simulink library "M160_control_lib"  (Simulink 7.8)
settings: Solver=FixedStepDiscrete  StartTime=0.0  StopTime=10.0  RelTol=1e-3
PreLoadFcn:
  | update_path
undefined symbols (not defined in the file): Egc_tiTEgasFilt, ehooks_medc17flex_devlib_io_block, Fmc_facKFuelMassCorr, Fmc_tiTFuelMassCorr, Itc_rpmEngSpdHyst, Itc_rpmEngSpdMax, Tvc_facDutycyclePIDLimitMax, Tvc_facDutycyclePIDLimitMin, Tvc_facKDutycycle, Tvc_tiTnDutycycle, Tvc_tiTvDutycycle
libraries: simulink x6
(part 2 of 2)

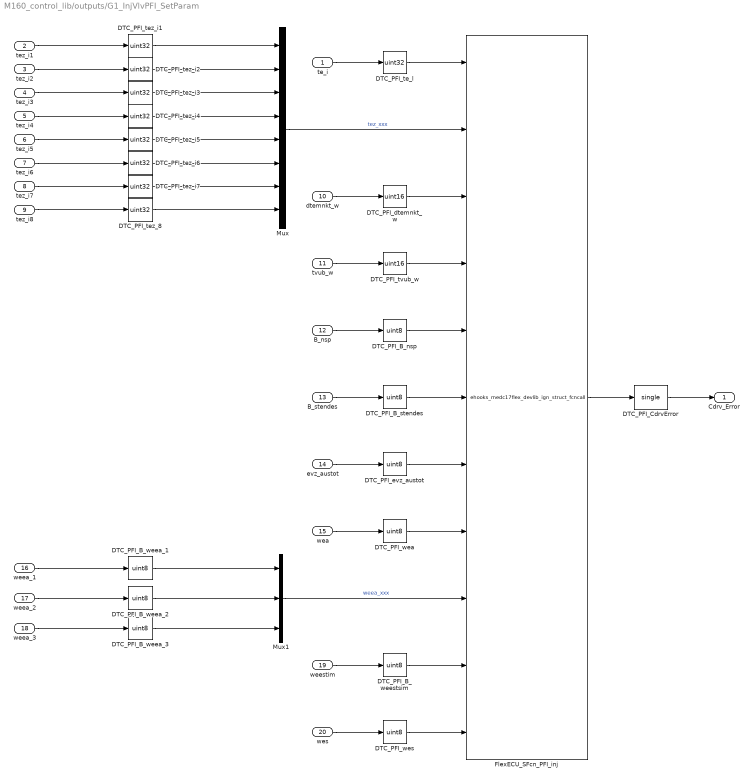
== system M160_control_lib/outputs/G1_InjVlvPFI_SetParam ==
  te_i : Inport
  tez_i1 : Inport  Port=2
  tez_i2 : Inport  Port=3
  tez_i3 : Inport  Port=4
  tez_i4 : Inport  Port=5
  tez_i5 : Inport  Port=6
  tez_i6 : Inport  Port=7
  tez_i7 : Inport  Port=8
  tez_i8 : Inport  Port=9
  dtemnkt_w : Inport  Port=10
  tvub_w : Inport  Port=11
  B_nsp : Inport  Port=12
  B_stendes : Inport  Port=13
  evz_austot : Inport  Port=14
  wea : Inport  Port=15
  weea_1 : Inport  Port=16
  weea_2 : Inport  Port=17
  weea_3 : Inport  Port=18
  weestim : Inport  Port=19
  wes : Inport  Port=20
  DTC_PFI_B_nsp : DataTypeConversion  OutDataTypeStr=uint8  RndMeth=Nearest
  DTC_PFI_B_stendes : DataTypeConversion  OutDataTypeStr=uint8  RndMeth=Nearest
  DTC_PFI_B_weea_1 : DataTypeConversion  OutDataTypeStr=uint8  RndMeth=Nearest
  DTC_PFI_B_weea_2 : DataTypeConversion  OutDataTypeStr=uint8
  DTC_PFI_B_weea_3 : DataTypeConversion  OutDataTypeStr=uint8  RndMeth=Nearest
  DTC_PFI_B_weestsim : DataTypeConversion  OutDataTypeStr=uint8  RndMeth=Nearest
  DTC_PFI_CdrvError : DataTypeConversion  OutDataTypeStr=single
  DTC_PFI_dtemnkt_w : DataTypeConversion  OutDataTypeStr=uint16  RndMeth=Nearest
  DTC_PFI_evz_austot : DataTypeConversion  OutDataTypeStr=uint8  RndMeth=Nearest
  DTC_PFI_te_l : DataTypeConversion  OutDataTypeStr=uint32  RndMeth=Nearest
  DTC_PFI_tez_8 : DataTypeConversion  OutDataTypeStr=uint32  RndMeth=Nearest
  DTC_PFI_tez_i{1..7} (7 alike) : DataTypeConversion  OutDataTypeStr=uint32  RndMeth=Nearest
  DTC_PFI_tvub_w : DataTypeConversion  OutDataTypeStr=uint16  RndMeth=Nearest
  DTC_PFI_wea : DataTypeConversion  OutDataTypeStr=uint8  RndMeth=Nearest
  DTC_PFI_wes : DataTypeConversion  OutDataTypeStr=uint8  RndMeth=Nearest
  FlexECU_SFcn_PFI_inj : S-Function  FunctionName=ehooks_medc17flex_devlib_ign_struct_fcncall  Parameters=NoInputPorts, NoOutputPorts, InputPortDataTypes, OutputPortDataTypes, CFunctionArgTypes, CFunctionName, StructMemberNames, StructTypeName, InputPortDataWidths, OutputPortDataWidths  EnableBusSupport=off  mask{NoInputPorts=11, NoOutputPorts=1, InputPortDataTypes=uint32, uint32, uint16, uint16,uint8,uint8,uint8,uint8,uint8,uint8,uint8, OutputPortDataTypes=uint8, CFunctionArgTypes=ret,val, refin, val,val,val,val,val, val, refin, val, val, CFunctionName=InjVlvPfi_SetParam, StructMemberNames=te_l,  tez_l, dtemnkt_w, tvub_w, B_nsp, B_stendes, evz_austot, wea, weea, weestsim, wes, StructTypeName=InjVlvPfiInterface_type, InputPortDataWidths=1,8,1,1,1,1,1,1,3,1,1, OutputPortDataWidths=1}
      mask prompts: NoInputPorts "Number of input ports"; NoOutputPorts "Number of output ports"; InputPortDataTypes "Input port data types"; OutputPortDataTypes "Output port data types"; CFunctionArgTypes "C function argument types"; CFunctionName "C function name"; StructMemberNames "Structure member names"; StructTypeName "Structure type name"; InputPortDataWidths "Input port widths"; OutputPortDataWidths "Output port widths"
      mask Display: disp('EHOOKS FlexECU\nDevLib Wrapper\nS-Function')
  Mux : Mux  Inputs=8
  Mux1 : Mux  Inputs=3
  Cdrv_Error : Outport
  wires:
  DTC_PFI_CdrvError/1 -> Cdrv_Error/1
  FlexECU_SFcn_PFI_inj/1 -> DTC_PFI_CdrvError/1
  DTC_PFI_B_stendes/1 -> FlexECU_SFcn_PFI_inj/6
  B_stendes/1 -> DTC_PFI_B_stendes/1
  DTC_PFI_B_nsp/1 -> FlexECU_SFcn_PFI_inj/5
  B_nsp/1 -> DTC_PFI_B_nsp/1
  DTC_PFI_tvub_w/1 -> FlexECU_SFcn_PFI_inj/4
  tvub_w/1 -> DTC_PFI_tvub_w/1
  DTC_PFI_dtemnkt_w/1 -> FlexECU_SFcn_PFI_inj/3
  dtemnkt_w/1 -> DTC_PFI_dtemnkt_w/1
  te_i/1 -> DTC_PFI_te_l/1
  DTC_PFI_evz_austot/1 -> FlexECU_SFcn_PFI_inj/7
  DTC_PFI_wea/1 -> FlexECU_SFcn_PFI_inj/8
  DTC_PFI_B_weestsim/1 -> FlexECU_SFcn_PFI_inj/10
  DTC_PFI_wes/1 -> FlexECU_SFcn_PFI_inj/11
  evz_austot/1 -> DTC_PFI_evz_austot/1
  wea/1 -> DTC_PFI_wea/1
  weea_1/1 -> DTC_PFI_B_weea_1/1
  weestim/1 -> DTC_PFI_B_weestsim/1
  wes/1 -> DTC_PFI_wes/1
  DTC_PFI_te_l/1 -> FlexECU_SFcn_PFI_inj/1
  tez_i1/1 -> DTC_PFI_tez_i1/1
  tez_i2/1 -> DTC_PFI_tez_i2/1
  tez_i3/1 -> DTC_PFI_tez_i3/1
  tez_i4/1 -> DTC_PFI_tez_i4/1
  tez_i5/1 -> DTC_PFI_tez_i5/1
  tez_i6/1 -> DTC_PFI_tez_i6/1
  tez_i7/1 -> DTC_PFI_tez_i7/1
  tez_i8/1 -> DTC_PFI_tez_8/1
  DTC_PFI_tez_i1/1 -> Mux/1
  DTC_PFI_tez_i2/1 -> Mux/2
  DTC_PFI_tez_i3/1 -> Mux/3
  DTC_PFI_tez_i4/1 -> Mux/4
  DTC_PFI_tez_i5/1 -> Mux/5
  DTC_PFI_tez_i6/1 -> Mux/6
  DTC_PFI_tez_i7/1 -> Mux/7
  DTC_PFI_tez_8/1 -> Mux/8
  Mux/1 -> FlexECU_SFcn_PFI_inj/2  "tez_xxx"
  weea_2/1 -> DTC_PFI_B_weea_2/1
  weea_3/1 -> DTC_PFI_B_weea_3/1
  DTC_PFI_B_weea_1/1 -> Mux1/1
  DTC_PFI_B_weea_2/1 -> Mux1/2
  DTC_PFI_B_weea_3/1 -> Mux1/3
  Mux1/1 -> FlexECU_SFcn_PFI_inj/9  "weea_xxx"

== system M160_control_lib/outputs/G1_Inj_Set_DEVE_forPFI ==
  B_desee : Inport
  B_sa : Inport  Port=2
  DTC_PFI_DEVE_Bdesee : DataTypeConversion  OutDataTypeStr=uint8  RndMeth=Nearest
  DTC_PFI_DEVE_Bsa : DataTypeConversion  OutDataTypeStr=uint8  RndMeth=Nearest
  DTC_PFI_DEVE_Bsa1 : DataTypeConversion  OutDataTypeStr=single
  FlexECU_SFcn_PFI_inj : S-Function  FunctionName=ehooks_medc17flex_devlib_ign_struct_fcncall  Parameters=NoInputPorts, NoOutputPorts, InputPortDataTypes, OutputPortDataTypes, CFunctionArgTypes, CFunctionName, StructMemberNames, StructTypeName, InputPortDataWidths, OutputPortDataWidths  EnableBusSupport=off  mask{NoInputPorts=2, NoOutputPorts=1, InputPortDataTypes=uint8,uint8, OutputPortDataTypes=uint8, CFunctionArgTypes=ret, val, val, CFunctionName=InjVlvDeve_SetParam, StructMemberNames=B_desee, B_sa, StructTypeName=InjVlvDeveInterface_type, InputPortDataWidths=1,1, OutputPortDataWidths=1}
      mask prompts: NoInputPorts "Number of input ports"; NoOutputPorts "Number of output ports"; InputPortDataTypes "Input port data types"; OutputPortDataTypes "Output port data types"; CFunctionArgTypes "C function argument types"; CFunctionName "C function name"; StructMemberNames "Structure member names"; StructTypeName "Structure type name"; InputPortDataWidths "Input port widths"; OutputPortDataWidths "Output port widths"
      mask Display: disp('EHOOKS FlexECU\nDevLib Wrapper\nS-Function')
  Cdrv_Error : Outport
  wires:
  DTC_PFI_DEVE_Bsa/1 -> FlexECU_SFcn_PFI_inj/2
  B_sa/1 -> DTC_PFI_DEVE_Bsa/1
  B_desee/1 -> DTC_PFI_DEVE_Bdesee/1
  DTC_PFI_DEVE_Bdesee/1 -> FlexECU_SFcn_PFI_inj/1
  FlexECU_SFcn_PFI_inj/1 -> DTC_PFI_DEVE_Bsa1/1
  DTC_PFI_DEVE_Bsa1/1 -> Cdrv_Error/1

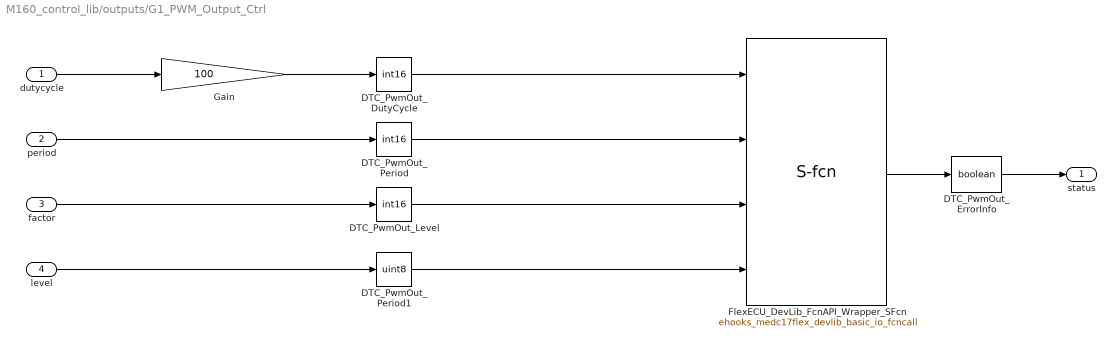
== system M160_control_lib/outputs/G1_PWM_Output_Ctrl ==
  dutycycle : Inport
  period : Inport  Port=2
  factor : Inport  Port=3
  level : Inport  Port=4
  DTC_PwmOut_DutyCycle : DataTypeConversion  OutDataTypeStr=int16  RndMeth=Nearest
  DTC_PwmOut_ErrorInfo : DataTypeConversion  OutDataTypeStr=boolean
  DTC_PwmOut_Level : DataTypeConversion  OutDataTypeStr=int16  RndMeth=Nearest
  DTC_PwmOut_Period : DataTypeConversion  OutDataTypeStr=int16  RndMeth=Nearest
  DTC_PwmOut_Period1 : DataTypeConversion  OutDataTypeStr=uint8  RndMeth=Nearest
  FlexECU_DevLib_FcnAPI_Wrapper_SFcn : S-Function  FunctionName=ehooks_medc17flex_devlib_basic_io_fcncall  Parameters=NoInputPorts, NoOutputPorts, InputPortDataTypes, OutputPortDataTypes, CFunctionArgTypes, CFunctionName, ChannelName  EnableBusSupport=off  mask{NoInputPorts=4, NoOutputPorts=1, InputPortDataTypes=int16,int16, int16, uint8, OutputPortDataTypes=uint8, CFunctionArgTypes=ret,val,val,val,val, CFunctionName=DevLib_Pwm_Out, ChannelName=<empty>}
      mask prompts: NoInputPorts "Number of input ports"; NoOutputPorts "Number of output ports"; InputPortDataTypes "Input port data types"; OutputPortDataTypes "Output port data types"; CFunctionArgTypes "C function argument types"; CFunctionName "C function name"; ChannelName "Channel (pin) name"
      mask Display: disp('EHOOKS FlexECU\nDevLib Wrapper\nS-Function')
  Gain : Gain  Gain=100
  status : Outport
  wires:
  Gain/1 -> DTC_PwmOut_DutyCycle/1
  dutycycle/1 -> Gain/1
  level/1 -> DTC_PwmOut_Period1/1
  DTC_PwmOut_Period1/1 -> FlexECU_DevLib_FcnAPI_Wrapper_SFcn/4
  FlexECU_DevLib_FcnAPI_Wrapper_SFcn/1 -> DTC_PwmOut_ErrorInfo/1
  period/1 -> DTC_PwmOut_Period/1
  factor/1 -> DTC_PwmOut_Level/1
  DTC_PwmOut_DutyCycle/1 -> FlexECU_DevLib_FcnAPI_Wrapper_SFcn/1
  DTC_PwmOut_Period/1 -> FlexECU_DevLib_FcnAPI_Wrapper_SFcn/2
  DTC_PwmOut_Level/1 -> FlexECU_DevLib_FcnAPI_Wrapper_SFcn/3
  DTC_PwmOut_ErrorInfo/1 -> status/1

== system M160_control_lib/outputs/G1_PwmOut_Get_error ==
  DTC_PwmOut_GetError : DataTypeConversion  OutDataTypeStr=single
  FlexECU_DevLib_FcnAPI_Wrapper_SFcn : S-Function  FunctionName=ehooks_medc17flex_devlib_basic_io_fcncall  Parameters=NoInputPorts, NoOutputPorts, InputPortDataTypes, OutputPortDataTypes, CFunctionArgTypes, CFunctionName, ChannelName  EnableBusSupport=off  mask{NoInputPorts=0, NoOutputPorts=1, InputPortDataTypes=, OutputPortDataTypes=uint8, CFunctionArgTypes=ret, CFunctionName=DevLib_PwmOut_GetError, ChannelName=<empty>}
      mask prompts: NoInputPorts "Number of input ports"; NoOutputPorts "Number of output ports"; InputPortDataTypes "Input port data types"; OutputPortDataTypes "Output port data types"; CFunctionArgTypes "C function argument types"; CFunctionName "C function name"; ChannelName "Channel (pin) name"
      mask Display: disp('EHOOKS FlexECU\nDevLib Wrapper\nS-Function')
  status : Outport
  wires:
  DTC_PwmOut_GetError/1 -> status/1
  FlexECU_DevLib_FcnAPI_Wrapper_SFcn/1 -> DTC_PwmOut_GetError/1

== system M160_control_lib/filters/PID_Limit_AWU/Limiter ==
  max : Inport
  in : Inport  Port=2
  min : Inport  Port=3
  Saturation Dynamic : simulink/Discontinuities/Saturation Dynamic  OutMin=[]  OutMax=[]  OutDataTypeStr=Inherit: Same as second input  OutDataType=fixdt(1, 16)  OutScaling=2^-10  DoSatur=off
  return : Outport
  wires:
  max/1 -> Saturation Dynamic/1
  in/1 -> Saturation Dynamic/2
  min/1 -> Saturation Dynamic/3
  Saturation Dynamic/1 -> return/1

== matlab function filters/LowpassT/MATLAB Function ==
  data: x output double; u input double; y output double
function [x,y]= fcn(u)
% initValue Test
if(u<0)
    y = 0;
else
    y = 1;
end

x = u;

== matlab function filters/LowpassT_Fcn/MATLAB Function ==
  data: u input double; y output double
function y = fcn(u)
% initValue Test
if(u<0)
    y = 0;
else
    y = 1;
end

== matlab function discontinuities/Accumulator/MATLAB Function ==
  data: u input double; y output double
function y = fcn(u)
% initValue Test
if(u<=0)
    y = 0;
else
    y = 1;
end

== matlab function discontinuities/Counter/MATLAB Function ==
  data: u input double; y output double
function y = fcn(u)
% initValue Test
if(u<=0)
    y = 0;
else
    y = 1;
end

== matlab function discontinuities/RSFlipFlop/MATLAB Function ==
  data: r input double; q output double; s input double
function q = fcn(r,s)
% FlipFlop
q = false;
if(r==true)
    q = false;
elseif(s==true)
    q = true;
end

== matlab function discontinuities/CounterEnabled/MATLAB Function ==
  data: u input double; y output double; v input double
function y = fcn(u,v)
% CounterEnabled Test
y = false;
if(u==true)
    y = false;
end
if(v==true)
    y = true;
end

== matlab function discontinuities/Integrator/MATLAB Function ==
  data: initEnable input double; out output double; initValue input double; enable input double; in input double
function out = fcn(initEnable,initValue,enable,in)
% Integrator Test
out = single(0.0);
if(initEnable==true)
    out = initValue;
end
if(enable==true)
    out = single(in);
end
